simulink model "LQR"  (Simulink 10.0)
settings: Solver=FixedStepAuto  StartTime=0.0  StopTime=50  FixedStep=0.001  RelTol=1e-3  EnableMultiTasking=on
values from neighbouring files (symbols this model uses):
  K = lqr(A_,B_,Q,R)    [LQR.m]
settings Model: Creator=HP-Computer  LastModifiedBy=Te
settings DataIOCC: LimitDataPoints=on  SignalLoggingSaveFormat=ModelDataLogs
settings OptimizationCC: ExpressionDepthLimit=2147483647
settings DebuggingCC: SolverPrmCheckMsg=warning  FcnCallInpInsideContextMsg=warning  StateNameClashWarn=warning
settings SFSimCC: SimParseCustomCode=off
settings GRTTargetCC: GeneratePreprocessorConditionals=Disable all
settings ConfigComp: CovExternalEMLEnable=off

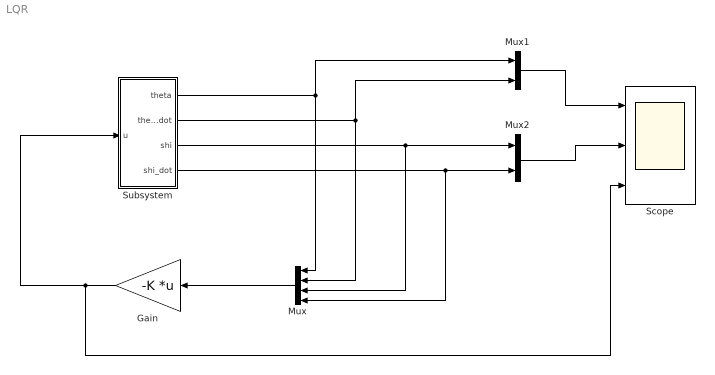
== system LQR ==
  Gain : Gain  Gain=-K  Multiplication=Matrix(K*u)
  Mux : Mux
  Mux1 : Mux  Inputs=2
  Mux2 : Mux  Inputs=2
  Scope : Scope  NumInputPorts=3
  Subsystem : Subsystem
  wires:
  Subsystem/1(theta) -> Mux/1, Mux1/1
  Subsystem/3(shi) -> Mux/3, Mux2/1
  Mux/1 -> Gain/1
  Gain/1 -> Subsystem/1(u), Scope/3
  Subsystem/2(theta_dot) -> Mux/2, Mux1/2
  Subsystem/4(shi_dot) -> Mux/4, Mux2/2
  Mux1/1 -> Scope/1
  Mux2/1 -> Scope/2

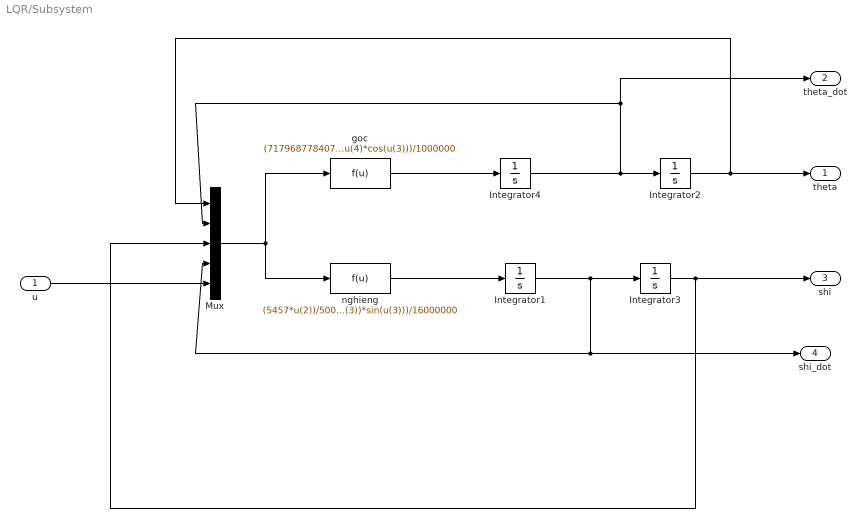
== system LQR/Subsystem ==
  u : Inport
  Integrator1 : Integrator  InitialCondition=0.001  UpperSaturationLimit=1  LowerSaturationLimit=-1
  Integrator2 : Integrator
  Integrator3 : Integrator  InitialCondition=pi/18  UpperSaturationLimit=1  LowerSaturationLimit=-1
  Integrator4 : Integrator  UpperSaturationLimit=1  LowerSaturationLimit=-1
  Mux : Mux  Inputs=5
  goc : Fcn  Expr=(7179687784074967909*u(5))/14073748835532800000 - (21506975204879888943*u(2))/14073748835532800000000 + (7179687784074967909*u(4))/7036874417766400000000 - (503253*sin(u(3)))/50000000 + (119393504331937137*u(4)*u(4)*sin(u(3)))/7205759403792793600 + (2304369*cos(u(3))*sin(u(3)))/4000000 - (261*u(5)*cos(u(3)))/2000 + (261*u(2)*cos(u(3)))/1000000 - (261*u(4)*cos(u(3)))/1000000
  nghieng : Fcn  Expr=(5457*u(2))/5000000 - (6807*u(5))/12500 - (6807*u(4))/6250000 + (119694753*sin(u(3)))/50000000 - (14877*u(4)*u(4)*sin(u(3)))/200000000 + (261*u(5)*cos(u(3)))/2000 - (783*u(2)*cos(u(3)))/2000000 + (261*u(4)*cos(u(3)))/1000000 + (68121*u(4)*u(4)*cos(u(3))*sin(u(3)))/16000000
  theta : Outport
  theta_dot : Outport  Port=2
  shi : Outport  Port=3
  shi_dot : Outport  Port=4
  wires:
  Integrator1/1 -> Integrator3/1, shi_dot/1, Mux/4
  Integrator4/1 -> Integrator2/1, theta_dot/1, Mux/2
  Mux/1 -> goc/1, nghieng/1
  nghieng/1 -> Integrator1/1
  goc/1 -> Integrator4/1
  u/1 -> Mux/5
  Integrator2/1 -> theta/1, Mux/1
  Integrator3/1 -> shi/1, Mux/3
